simulink model "number1"  (R2022b)
settings: Solver=VariableStepAuto  StartTime=0.0  StopTime=100.0  RelTol=1e-3
settings Model: Creator=lenovo  LastModifiedBy=acer
settings DataIOCC: ReturnWorkspaceOutputs=off
settings ModelReferenceCC: EnableRefExpFcnMdlSchedulingChecks=on

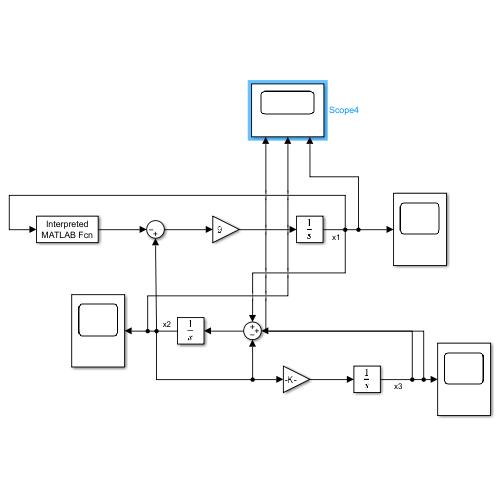
[thumbnail: Simulink's stored preview of the top-level diagram]
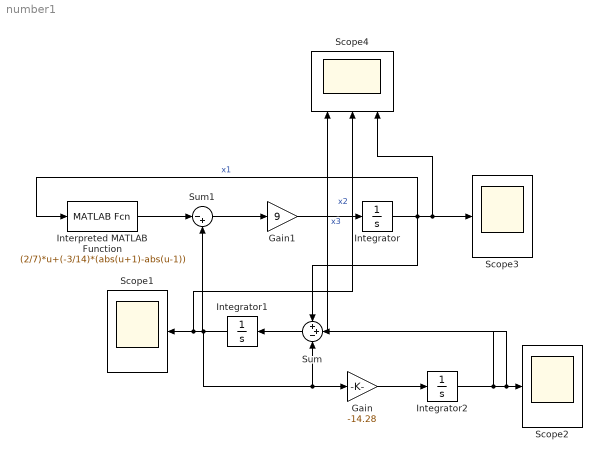
== system number1 ==
  Gain : Gain  Gain=-14.28
  Gain1 : Gain  Gain=9
  Integrator : Integrator  InitialCondition=1
  Integrator1 : Integrator  InitialCondition=2
  Integrator2 : Integrator  InitialCondition=3
  Interpreted MATLAB Function : MATLABFcn  MATLABFcn=(2/7)*u+(-3/14)*(abs(u+1)-abs(u-1))
  Scope1 : Scope
  Scope2 : Scope
  Scope3 : Scope
  Scope4 : Scope  NumInputPorts=3
  Sum : Sum  Inputs=++-
  Sum1 : Sum  Inputs=|-+
  wires:
  Integrator/1 -> Scope3/1, Scope4/3, Interpreted MATLAB Function/1, Sum/1  "x1"
  Integrator1/1 -> Scope4/2, Scope1/1, Gain/1, Sum/3, Sum1/2  "x2"
  Gain/1 -> Integrator2/1
  Integrator2/1 -> Scope4/1, Scope2/1, Sum/2  "x3"
  Sum/1 -> Integrator1/1
  Sum1/1 -> Gain1/1
  Gain1/1 -> Integrator/1
  Interpreted MATLAB Function/1 -> Sum1/1
